simulink model "es5_ACPC_sim"  (R2022b)
settings: Solver=VariableStepAuto  StartTime=0.0  StopTime=10.0  RelTol=1e-3
values from neighbouring files (symbols this model uses):
  A = [-a b;c -d]    [ES5.m]
  alfa = -inv(C*inv(A-B*K2)*B)    [ES5.m]
  B = [1;1]    [ES5.m]
  C = [1 1]    [ES5.m]
  K1 = place(A,B,avalD)    [ES5.m]
settings Model: Creator=claudio  LastModifiedBy=claudio

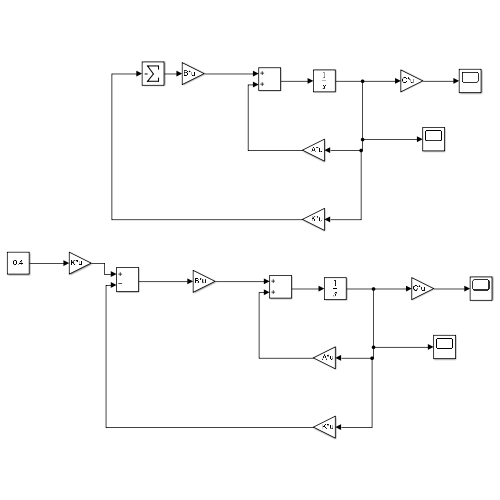
[thumbnail: Simulink's stored preview of the top-level diagram]
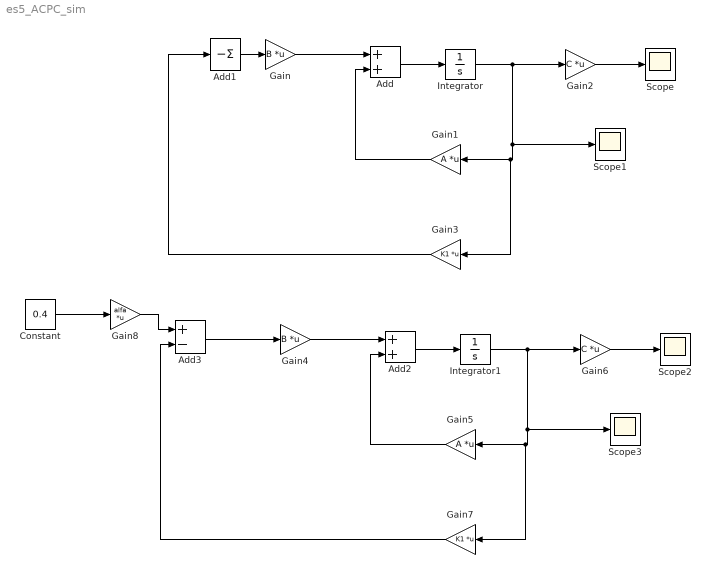
== system es5_ACPC_sim ==
  Add : Sum
  Add1 : Sum  Inputs=-
  Add2 : Sum
  Add3 : Sum  Inputs=+-
  Constant : Constant  Value=0.4
  Gain : Gain  Gain=B  Multiplication=Matrix(K*u)
  Gain1 : Gain  Gain=A  Multiplication=Matrix(K*u)
  Gain2 : Gain  Gain=C  Multiplication=Matrix(K*u)
  Gain3 : Gain  Gain=K1  Multiplication=Matrix(K*u)
  Gain4 : Gain  Gain=B  Multiplication=Matrix(K*u)
  Gain5 : Gain  Gain=A  Multiplication=Matrix(K*u)
  Gain6 : Gain  Gain=C  Multiplication=Matrix(K*u)
  Gain7 : Gain  Gain=K1  Multiplication=Matrix(K*u)
  Gain8 : Gain  Gain=alfa  Multiplication=Matrix(K*u)
  Integrator : Integrator  InitialCondition=[0.5;0.3]
  Integrator1 : Integrator  InitialCondition=[0.5;0.3]
  Scope{,1..3} (4 alike) : Scope
  wires:
  Add/1 -> Integrator/1
  Gain/1 -> Add/1
  Gain1/1 -> Add/2
  Integrator/1 -> Scope1/1, Gain3/1, Gain1/1, Gain2/1
  Add1/1 -> Gain/1
  Gain3/1 -> Add1/1
  Gain2/1 -> Scope/1
  Add3/1 -> Gain4/1
  Add2/1 -> Integrator1/1
  Gain5/1 -> Add2/2
  Gain4/1 -> Add2/1
  Integrator1/1 -> Scope3/1, Gain7/1, Gain5/1, Gain6/1
  Gain6/1 -> Scope2/1
  Gain7/1 -> Add3/2
  Gain8/1 -> Add3/1
  Constant/1 -> Gain8/1
